simulink model "test_loop_interno"  (R2023a)
settings: Solver=FixedStepAuto  StartTime=0.0  StopTime=10  FixedStep=0.00001  RelTol=1e-3
undefined symbols (not defined in the file or in its folder): G, Gz, pi_pos
libraries: simulink x4
settings Model: Creator=edoar  LastModifiedBy=edoar
settings SolverCC: AlgebraicLoopSolver=TrustRegion
settings DebuggingCC: UnconnectedInputMsg=warning  UnconnectedOutputMsg=warning  UnconnectedLineMsg=warning
settings ModelReferenceCC: EnableRefExpFcnMdlSchedulingChecks=on

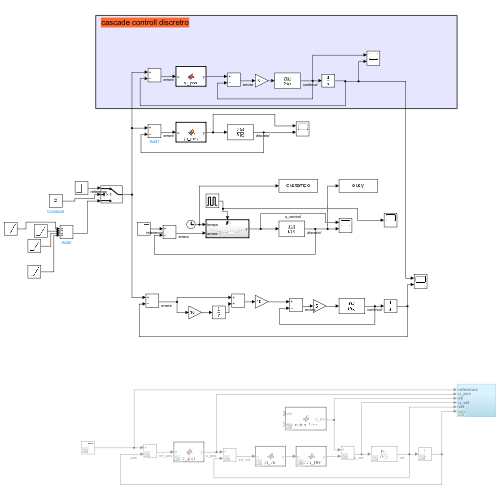
[thumbnail: Simulink's stored preview of the top-level diagram]
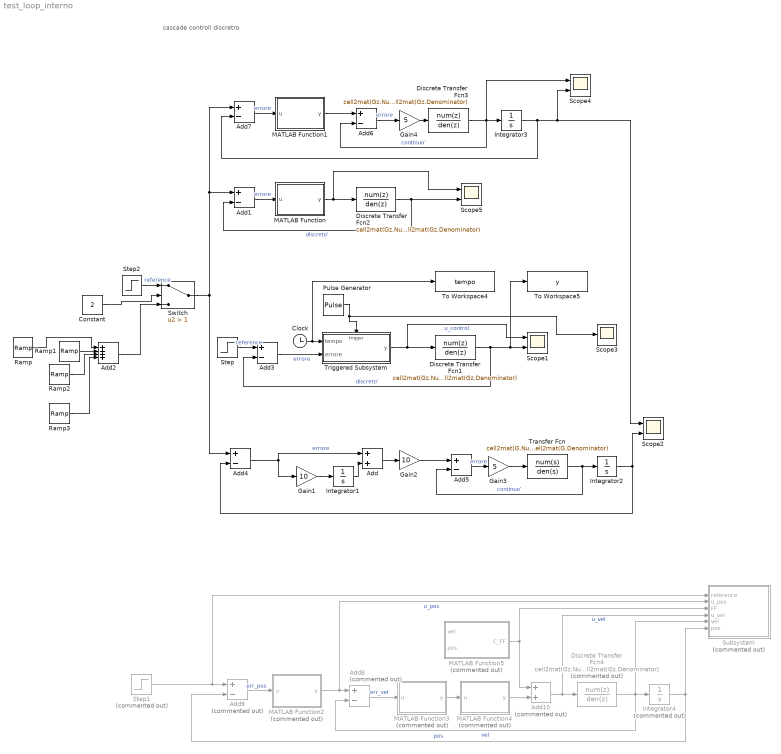
== system test_loop_interno ==
  note: cascade controll discretro
  Add : Sum
  Add{1,3..7} (6 alike) : Sum  Inputs=+-
  Add10 : Sum  Commented=on
  Add2 : Sum  Inputs=++++
  Add8 : Sum  Commented=on  Inputs=+-
  Add9 : Sum  Commented=on  Inputs=+-
  Clock : Clock
  Constant : Constant  Value=2
  Discrete Transfer Fcn1 : DiscreteTransferFcn  Numerator=cell2mat(Gz.Numerator)  Denominator=cell2mat(Gz.Denominator)  SampleTime=0.001
  Discrete Transfer Fcn2 : DiscreteTransferFcn  Numerator=cell2mat(Gz.Numerator)  Denominator=cell2mat(Gz.Denominator)  SampleTime=0.001
  Discrete Transfer Fcn3 : DiscreteTransferFcn  Numerator=cell2mat(Gz.Numerator)  Denominator=cell2mat(Gz.Denominator)  SampleTime=0.001
  Discrete Transfer Fcn4 : DiscreteTransferFcn  Commented=on  Numerator=cell2mat(Gz.Numerator)  Denominator=cell2mat(Gz.Denominator)  SampleTime=0.001
  Gain1 : Gain  Gain=10
  Gain2 : Gain  Gain=10
  Gain3 : Gain  Gain=5
  Gain4 : Gain  Gain=5
  Integrator1 : Integrator
  Integrator2 : Integrator
  Integrator3 : Integrator
  Integrator4 : Integrator  Commented=on
  MATLAB Function : MATLAB Function  TreatAsAtomicUnit=on  SystemSampleTime=0.001
  MATLAB Function1 : MATLAB Function  TreatAsAtomicUnit=on  SystemSampleTime=0.001
  MATLAB Function2 : MATLAB Function  Commented=on  TreatAsAtomicUnit=on  SystemSampleTime=0.001
  MATLAB Function3 : MATLAB Function  Commented=on  TreatAsAtomicUnit=on  SystemSampleTime=0.001
  MATLAB Function4 : MATLAB Function  Commented=on  TreatAsAtomicUnit=on  SystemSampleTime=0.001
  MATLAB Function5 : MATLAB Function  Commented=on  TreatAsAtomicUnit=on  SystemSampleTime=0.001
  Pulse Generator : DiscretePulseGenerator  PulseType=Time based  Period=0.001  PulseWidth=50
  Ramp : simulink/Sources/Ramp  slope=1  start=0  InitialOutput=0
  Ramp1 : simulink/Sources/Ramp  slope=-1  start=1  InitialOutput=0
  Ramp2 : simulink/Sources/Ramp  slope=-1  start=3  InitialOutput=0
  Ramp3 : simulink/Sources/Ramp  slope=1  start=4  InitialOutput=0
  Scope{1..2,4..5} (4 alike) : Scope  NumInputPorts=2
  Scope3 : Scope
  Step : Step  Time=0  SampleTime=0
  Step1 : Step  Commented=on  SampleTime=0
  Step2 : Step  Time=0  SampleTime=0
  Subsystem : Subsystem  Commented=on
  Switch : Switch  Criteria=u2 > Threshold  Threshold=1  SaturateOnIntegerOverflow=off  InputSameDT=off
  To Workspace4 : ToWorkspace  VariableName=tempo  SaveFormat=Timeseries  SampleTime=-1
  To Workspace5 : ToWorkspace  VariableName=y  SaveFormat=Timeseries  SampleTime=-1
  Transfer Fcn : TransferFcn  Numerator=cell2mat(G.Numerator)  Denominator=cell2mat(G.Denominator)
  Triggered Subsystem : Subsystem  TreatAsAtomicUnit=on
  wires:
  Pulse Generator/1 -> Triggered Subsystem/Trigger, Scope3/1
  Step/1 -> Add3/1  "reference"
  Triggered Subsystem/1(y) -> Scope1/1, Discrete Transfer Fcn1/1  "u_control"
  Discrete Transfer Fcn1/1 -> To Workspace5/1, Scope1/2, Add3/2  "discreto'"
  Add3/1 -> Triggered Subsystem/2(errore)  "errore"
  Clock/1 -> To Workspace4/1, Triggered Subsystem/1(tempo)
  Gain1/1 -> Integrator1/1
  Integrator1/1 -> Add/2
  Add4/1 -> Gain1/1, Add/1  "errore"
  Add/1 -> Gain2/1
  Add1/1 -> MATLAB Function/1(u)  "errore"
  MATLAB Function/1(y) -> Scope5/1, Discrete Transfer Fcn2/1
  Discrete Transfer Fcn2/1 -> Scope5/2, Add1/2  "discreto'"
  Ramp/1 -> Add2/1
  Ramp1/1 -> Add2/2
  Ramp2/1 -> Add2/3
  Ramp3/1 -> Add2/4
  Add2/1 -> Switch/3
  Step2/1 -> Switch/1  "reference"
  Switch/1 -> Add4/1, Add7/1, Add1/1
  Gain2/1 -> Add5/1
  Add5/1 -> Gain3/1  "errore"
  Gain3/1 -> Transfer Fcn/1
  Transfer Fcn/1 -> Add5/2, Integrator2/1  "continuo'"
  Integrator2/1 -> Scope2/2, Add4/2
  MATLAB Function1/1(y) -> Add6/1
  Add6/1 -> Gain4/1  "errore"
  Discrete Transfer Fcn3/1 -> Add6/2, Scope4/1, Integrator3/1  "continuo'"
  Add7/1 -> MATLAB Function1/1(u)  "errore"
  Integrator3/1 -> Scope4/2, Scope2/1, Add7/2
  Gain4/1 -> Discrete Transfer Fcn3/1
  Constant/1 -> Switch/2
  Add10/1 -> Subsystem/4(u_vel), Discrete Transfer Fcn4/1  "u_vel"
  Discrete Transfer Fcn4/1 -> Subsystem/5(vel), Add8/2, Integrator4/1  "vel"
  Integrator4/1 -> Add9/2, Subsystem/6(pos)  "pos"
  Add9/1 -> MATLAB Function2/1(u)  "err_pos"
  MATLAB Function2/1(y) -> Subsystem/2(u_pos), Add8/1  "u_pos"
  Add8/1 -> MATLAB Function3/1(u)  "err_vel"
  MATLAB Function3/1(y) -> MATLAB Function4/1(u)
  MATLAB Function4/1(y) -> Add10/2
  MATLAB Function5/1(C_FF) -> Subsystem/3(FF), Add10/1
  Step1/1 -> Subsystem/1(reference), Add9/1

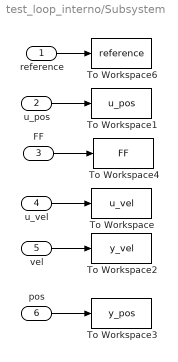
== system test_loop_interno/Subsystem ==
  reference : Inport
  u_pos : Inport  Port=2
  FF : Inport  Port=3
  u_vel : Inport  Port=4
  vel : Inport  Port=5
  pos : Inport  Port=6
  To Workspace : ToWorkspace  VariableName=u_vel  SaveFormat=Timeseries  SampleTime=-1
  To Workspace1 : ToWorkspace  VariableName=u_pos  SaveFormat=Timeseries  SampleTime=-1
  To Workspace2 : ToWorkspace  VariableName=y_vel  SaveFormat=Timeseries  SampleTime=-1
  To Workspace3 : ToWorkspace  VariableName=y_pos  SaveFormat=Timeseries  SampleTime=-1
  To Workspace4 : ToWorkspace  VariableName=FF  SaveFormat=Timeseries  SampleTime=-1
  To Workspace6 : ToWorkspace  VariableName=reference  SaveFormat=Timeseries  SampleTime=-1
  wires:
  reference/1 -> To Workspace6/1
  u_vel/1 -> To Workspace/1
  vel/1 -> To Workspace2/1
  pos/1 -> To Workspace3/1
  u_pos/1 -> To Workspace1/1
  FF/1 -> To Workspace4/1

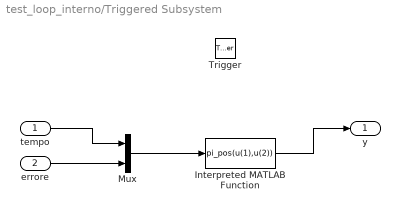
== system test_loop_interno/Triggered Subsystem ==
  tempo : Inport
  errore : Inport  Port=2
  Trigger : TriggerPort  VariantControl=Variant
  Interpreted MATLAB Function : MATLABFcn  MATLABFcn=pi_pos(u(1),u(2))
  Mux : Mux  Inputs=2
  y : Outport
  wires:
  tempo/1 -> Mux/1
  errore/1 -> Mux/2
  Mux/1 -> Interpreted MATLAB Function/1
  Interpreted MATLAB Function/1 -> y/1

== matlab function test_loop_interno/MATLAB Function ==
  data: u input; y output
function y = pi_pos(u)
    Kp = 10;
    Ki = 10;
    persistent ym1  um1
    if isempty(ym1)%
        ym1 = 0.;
        um1 = 0;
        y = 0;
    else
        y_now = ym1+Kp*((1+(Ki*0.001))*u-um1);
        um1 = u;
        ym1 = y_now;
        y = y_now;
    end
end

== matlab function test_loop_interno/MATLAB Function2 ==
  data: u input; y output
function y = pi_pos(u)
    Kp = 10;
    Ki = 10;
    persistent ym1  um1
    if isempty(ym1)%
        ym1 = 0.;
        um1 = 0;
        y = 0;
    else
        y_now = ym1+Kp*((1+(Ki*0.001))*u-um1);
        um1 = u;
        ym1 = y_now;
        y = y_now;
    end
end

== matlab function test_loop_interno/MATLAB Function3 ==
  data: u input; y output
function y = pi_vel(u)
    Kp = 10;
    Ki = 10;
    persistent ym1  um1
    if isempty(ym1)%
        ym1 = 0.;
        um1 = 0;
        y = 0;
    else
        y =Kp*u;
    end
end

== matlab function test_loop_interno/MATLAB Function4 ==
  data: u input; y output
function y = notch_filter(u)
    Kp = 10;
    Ki = 10;
    persistent ym1  um1
    if isempty(ym1)%
        ym1 = 0.;
        um1 = 0;
        y = 0;
    else
        y=u
    end
end

== matlab function test_loop_interno/MATLAB Function5 ==
  data: vel input; C_FF output; pos input
function C_FF= notch_filter(vel,pos)
    Kp = 10;
    Ki = 10;
    persistent ym1  um1
    if isempty(ym1)%
        ym1 = 0.;
        um1 = 0;
        y = 0;
    else
        0
    end
end

== matlab function test_loop_interno/MATLAB Function1 ==
  data: u input; y output
function y = pi_pos(u)
    Kp = 10;
    Ki = 10;
    persistent ym1  um1
    if isempty(ym1)%
        ym1 = 0.;
        um1 = 0;
        y = 0;
    else
        y_now = ym1+Kp*((1+(Ki*0.001))*u-um1);
        um1 = u;
        ym1 = y_now;
        y = y_now;
    end
end
